simulink model "APP_Logic_System"  (R2021a)
settings: Solver=FixedStepDiscrete  StartTime=0.0  StopTime=10.0  RelTol=1e-3
settings Model: Creator=lenovo  LastModifiedBy=lenovo
settings OptimizationCC: DefaultParameterBehavior=Inlined  UseDivisionForNetSlopeComputation=on  GainParamInheritBuiltInType=on  UseFloatMulNetSlope=on  InlineInvariantSignals=on  PassReuseOutputArgsAs=Individual arguments  ZeroExternalMemoryAtStartup=off  ZeroInternalMemoryAtStartup=off  NoFixptDivByZeroProtection=on  EfficientFloat2IntCast=on  LifeSpan=1  OptimizeBlockOrder=speed  DifferentSizesBufferReuse=on  EfficientTunableParamExpr=on
settings DebuggingCC: ParameterTunabilityLossMsg=error
settings HardwareCC: ProdBitPerPointer=32  ProdBitPerSizeT=32  ProdBitPerPtrDiffT=32  ProdLargestAtomicInteger=Long  ProdLargestAtomicFloat=Double  ProdWordSize=32  ProdLongLongMode=on  ProdHWDeviceType=ARM Compatible->ARM Cortex-M
settings SFSimCC: MATLABDynamicMemAlloc=off
settings RTWCC: SystemTargetFile=ert.tlc  TemplateMakefile=ert_default_tmf
settings CodeAppCC: ForceParamTrailComments=on  IgnoreCustomStorageClasses=off  OperatorAnnotations=on  SimulinkDataObjDesc=on  SFDataObjDesc=on  CustomSymbolStrGlobalVar=rt$N$M  CustomSymbolStrType=$N$M  CustomSymbolStrFcn=$N$M$F  CustomSymbolStrMacro=$N$M  InsertBlockDesc=on
settings ERTTargetCC: TargetLangStandard=C99 (ISO)  GenerateSampleERTMain=on  IncludeMdlTerminateFcn=off  CombineSignalStateStructs=on  SuppressErrorStatus=on  SupportAbsoluteTime=off  SupportComplex=off  InlinedParameterPlacement=NonHierarchical  ERTCustomFileTemplate=example_file_process.tlc  ERTFilePackagingFormat=CompactWithDataFile

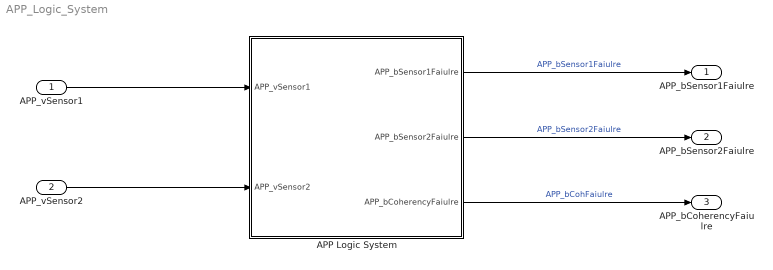
== system APP_Logic_System ==
  APP_vSensor1 : Inport
  APP_vSensor2 : Inport  Port=2
  APP Logic System : Subsystem  TreatAsAtomicUnit=on
      settings: RTWSystemCode=Nonreusable function
  APP_bSensor1Faiulre : Outport
  APP_bSensor2Faiulre : Outport  Port=2
  APP_bCoherencyFaiulre : Outport  Port=3
  wires:
  APP_vSensor1/1 -> APP Logic System/1(APP_vSensor1)
  APP Logic System/3(APP_bCoherencyFaiulre) -> APP_bCoherencyFaiulre/1  "APP_bCohFaiulre"
  APP Logic System/1(APP_bSensor1Faiulre) -> APP_bSensor1Faiulre/1  "APP_bSensor1Faiulre"
  APP_vSensor2/1 -> APP Logic System/2(APP_vSensor2)
  APP Logic System/2(APP_bSensor2Faiulre) -> APP_bSensor2Faiulre/1  "APP_bSensor2Faiulre"

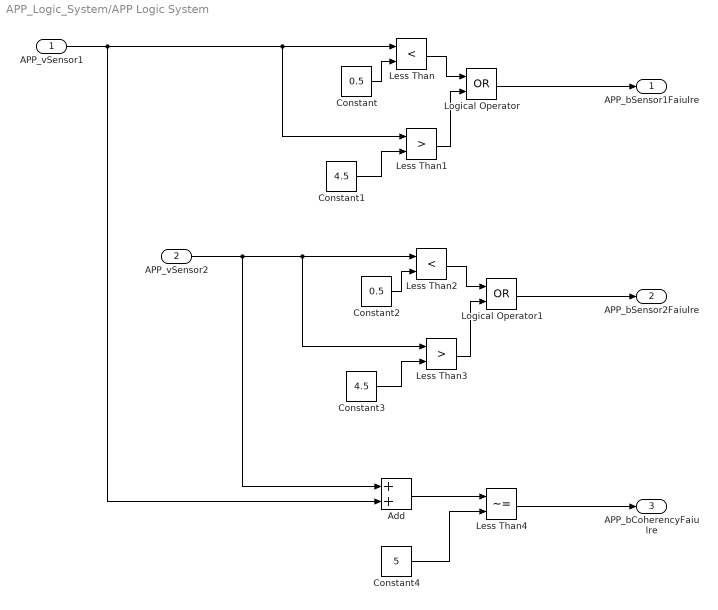
== system APP_Logic_System/APP Logic System ==
  APP_vSensor1 : Inport
  APP_vSensor2 : Inport  Port=2
  Add : Sum
  Constant : Constant  Value=0.5
  Constant1 : Constant  Value=4.5
  Constant2 : Constant  Value=0.5
  Constant3 : Constant  Value=4.5
  Constant4 : Constant  Value=5
  Less Than : RelationalOperator  Operator=<  OutDataTypeStr=boolean  RndMeth=Simplest
  Less Than1 : RelationalOperator  Operator=>  OutDataTypeStr=boolean  RndMeth=Simplest
  Less Than2 : RelationalOperator  Operator=<  OutDataTypeStr=boolean  RndMeth=Simplest
  Less Than3 : RelationalOperator  Operator=>  OutDataTypeStr=boolean  RndMeth=Simplest
  Less Than4 : RelationalOperator  Operator=~=  OutDataTypeStr=boolean  RndMeth=Simplest
  Logical Operator : Logic  Operator=OR  AllPortsSameDT=off  OutDataTypeStr=boolean
  Logical Operator1 : Logic  Operator=OR  AllPortsSameDT=off  OutDataTypeStr=boolean
  APP_bSensor1Faiulre : Outport
  APP_bSensor2Faiulre : Outport  Port=2
  APP_bCoherencyFaiulre : Outport  Port=3
  wires:
  Constant/1 -> Less Than/2
  APP_vSensor1/1 -> Add/2, Less Than1/1, Less Than/1
  APP_vSensor2/1 -> Add/1, Less Than3/1, Less Than2/1
  Add/1 -> Less Than4/1
  Less Than3/1 -> Logical Operator1/2
  Constant1/1 -> Less Than1/2
  Less Than/1 -> Logical Operator/1
  Less Than1/1 -> Logical Operator/2
  Logical Operator1/1 -> APP_bSensor2Faiulre/1
  Less Than2/1 -> Logical Operator1/1
  Less Than4/1 -> APP_bCoherencyFaiulre/1
  Constant3/1 -> Less Than3/2
  Constant2/1 -> Less Than2/2
  Constant4/1 -> Less Than4/2
  Logical Operator/1 -> APP_bSensor1Faiulre/1
